simulink subsystem "BiasUpdate"  (R2021a)
settings: Solver=VariableStepAuto  StartTime=0.0  StopTime=10.0  RelTol=1e-3
undefined symbols (not defined in the file): imu1, imu2, imu3, imu4
settings Model: Creator=Laura  LastModifiedBy=Laura

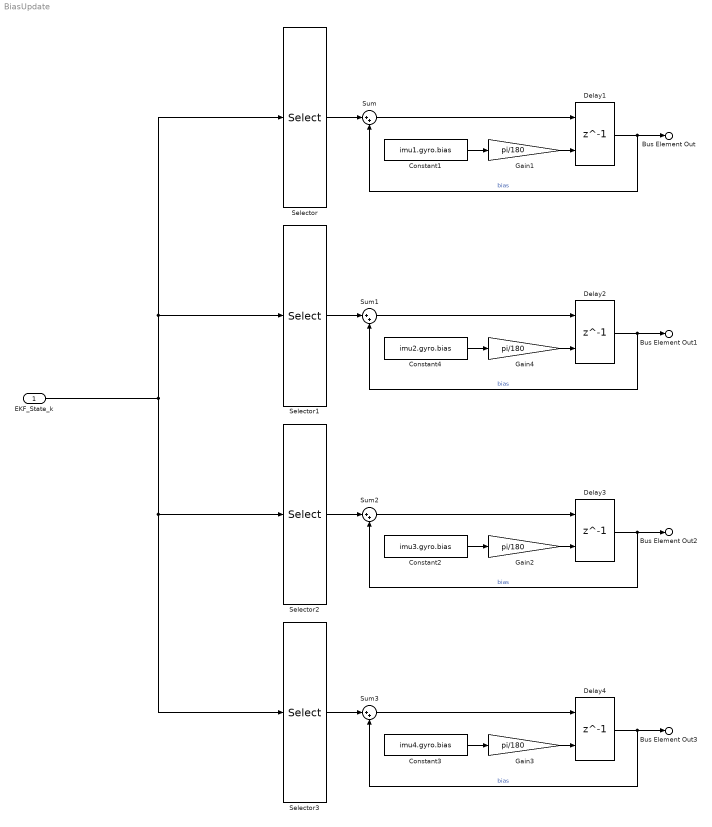
== system BiasUpdate ==
  EKF_State_k : Inport
  Constant1 : Constant  Value=imu1.gyro.bias
  Constant2 : Constant  Value=imu3.gyro.bias
  Constant3 : Constant  Value=imu4.gyro.bias
  Constant4 : Constant  Value=imu2.gyro.bias
  Delay{1..4} (4 alike) : Delay  DelayLength=1  InitialConditionSource=Input port
      settings: InputPortMap=u0,p4
  Gain{1..4} (4 alike) : Gain  Gain=pi/180
  Selector : Selector  InputPortWidth=24  IndexOptions=Index vector (dialog)  Indices=[4 5 6]  OutputSizes=1
  Selector1 : Selector  InputPortWidth=24  IndexOptions=Index vector (dialog)  Indices=[10 11 12]  OutputSizes=1
  Selector2 : Selector  InputPortWidth=24  IndexOptions=Index vector (dialog)  Indices=[16 17 18]  OutputSizes=1
  Selector3 : Selector  InputPortWidth=24  IndexOptions=Index vector (dialog)  Indices=[22 23 24]  OutputSizes=1
  Sum{,1..3} (4 alike) : Sum  Inputs=|++
  Bus Element Out : Outport  PortName=EKFBias  Element=bias_B1
  Bus Element Out1 : Outport  PortName=EKFBias  Element=bias_B2
  Bus Element Out2 : Outport  PortName=EKFBias  Element=bias_B3
  Bus Element Out3 : Outport  PortName=EKFBias  Element=bias_B4
  wires:
  Gain3/1 -> Delay4/2
  Selector3/1 -> Sum3/1
  Sum3/1 -> Delay4/1
  Constant3/1 -> Gain3/1
  Delay4/1 -> Bus Element Out3/1, Sum3/2  "bias"
  Gain2/1 -> Delay3/2
  Selector2/1 -> Sum2/1
  Sum2/1 -> Delay3/1
  Constant2/1 -> Gain2/1
  Delay3/1 -> Bus Element Out2/1, Sum2/2  "bias"
  Gain4/1 -> Delay2/2
  Selector1/1 -> Sum1/1
  Sum1/1 -> Delay2/1
  Constant4/1 -> Gain4/1
  Delay2/1 -> Bus Element Out1/1, Sum1/2  "bias"
  Gain1/1 -> Delay1/2
  Delay1/1 -> Bus Element Out/1, Sum/2  "bias"
  Sum/1 -> Delay1/1
  Constant1/1 -> Gain1/1
  Selector/1 -> Sum/1
  EKF_State_k/1 -> Selector/1, Selector1/1, Selector2/1, Selector3/1
